simulink model "uav_1"  (R2015b)
settings: Solver=ode4  StartTime=0.0  StopTime=10  FixedStep=0.05  RelTol=1e-3
undefined symbols (not defined in the file): ctrsel, dphi_init, dpsi_init, dthe_init, dx_init, dy_init, dz_init, g, Jx, Jy, Jz, K1, K2, K3, K4, K5, K6, kt, l, m, omega1, omega2, omega3, omega4, phi_init, psi_init, the_init, x_init, y_init, z_init
settings Model: Creator=Administrator  LastModifiedBy=Administrator

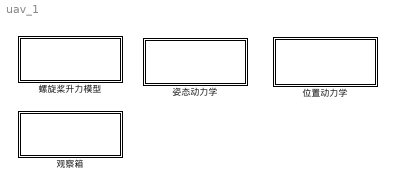
== system uav_1 ==
  位置动力学 : Subsystem
  姿态动力学 : Subsystem
  螺旋桨升力模型 : Subsystem
  观察箱 : Subsystem

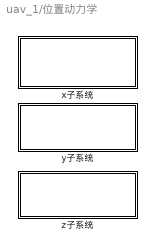
== system uav_1/位置动力学 ==
  x子系统 : Subsystem
  y子系统 : Subsystem
  z子系统 : Subsystem

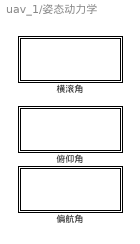
== system uav_1/姿态动力学 ==
  俯仰角 : Subsystem
  偏航角 : Subsystem
  横滚角 : Subsystem

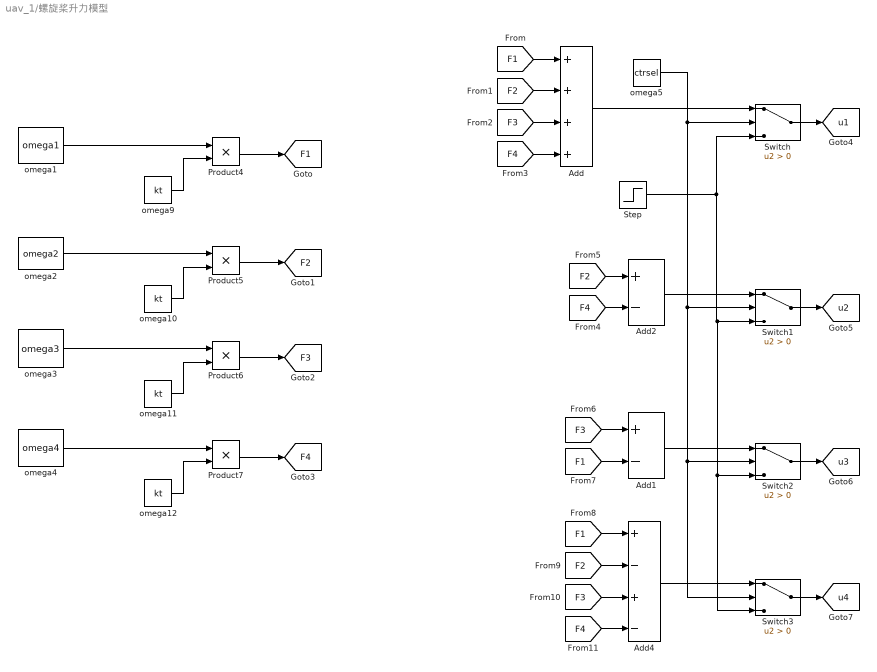
== system uav_1/螺旋桨升力模型 ==
  Add : Sum  Inputs=++++
  Add1 : Sum  Inputs=+-
  Add2 : Sum  Inputs=+-
  Add4 : Sum  Inputs=+-+-
  Product{4..7} (4 alike) : Product
  Step : Step  After=400  SampleTime=0
  Switch{,1..3} (4 alike) : Switch  Criteria=u2 > Threshold
  omega1 : Constant  Value=omega1
  omega{9..12} (4 alike) : Constant  Value=kt
  omega2 : Constant  Value=omega2
  omega3 : Constant  Value=omega3
  omega4 : Constant  Value=omega4
  omega5 : Constant  Value=ctrsel
  tag scope: F1=global, F2=global, F3=global, F4=global, u1=global, u2=global, u3=global, u4=global
  wires:
  [F3] -> Add/3
  [F4] -> Add/4
  [F1] -> Add1/2
  [F3] -> Add1/1
  [F2] -> Add/2
  [F1] -> Add/1
  [F1] -> Add4/1
  [F2] -> Add4/2
  [F3] -> Add4/3
  [F4] -> Add4/4
  [F4] -> Add2/2
  [F2] -> Add2/1
  omega1/1 -> Product4/1
  omega9/1 -> Product4/2
  Product4/1 -> [F1]
  omega2/1 -> Product5/1
  omega10/1 -> Product5/2
  Product5/1 -> [F2]
  omega3/1 -> Product6/1
  omega11/1 -> Product6/2
  Product6/1 -> [F3]
  omega4/1 -> Product7/1
  omega12/1 -> Product7/2
  Product7/1 -> [F4]
  omega5/1 -> Switch/2, Switch1/2, Switch2/2, Switch3/2
  Step/1 -> Switch/3, Switch3/3, Switch2/3, Switch1/3
  Add/1 -> Switch/1
  Add2/1 -> Switch1/1
  Add1/1 -> Switch2/1
  Add4/1 -> Switch3/1
  Switch/1 -> [u1]
  Switch1/1 -> [u2]
  Switch2/1 -> [u3]
  Switch3/1 -> [u4]

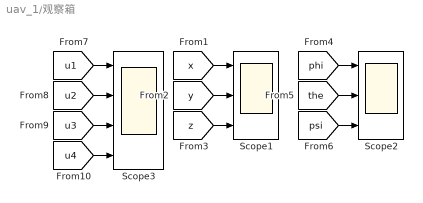
== system uav_1/观察箱 ==
  Scope1 : Scope  NumInputPorts=3
  Scope2 : Scope  NumInputPorts=3
  Scope3 : Scope  NumInputPorts=4
  wires:
  [x] -> Scope1/1
  [y] -> Scope1/2
  [z] -> Scope1/3
  [phi] -> Scope2/1
  [the] -> Scope2/2
  [psi] -> Scope2/3
  [u1] -> Scope3/1
  [u2] -> Scope3/2
  [u3] -> Scope3/3
  [u4] -> Scope3/4

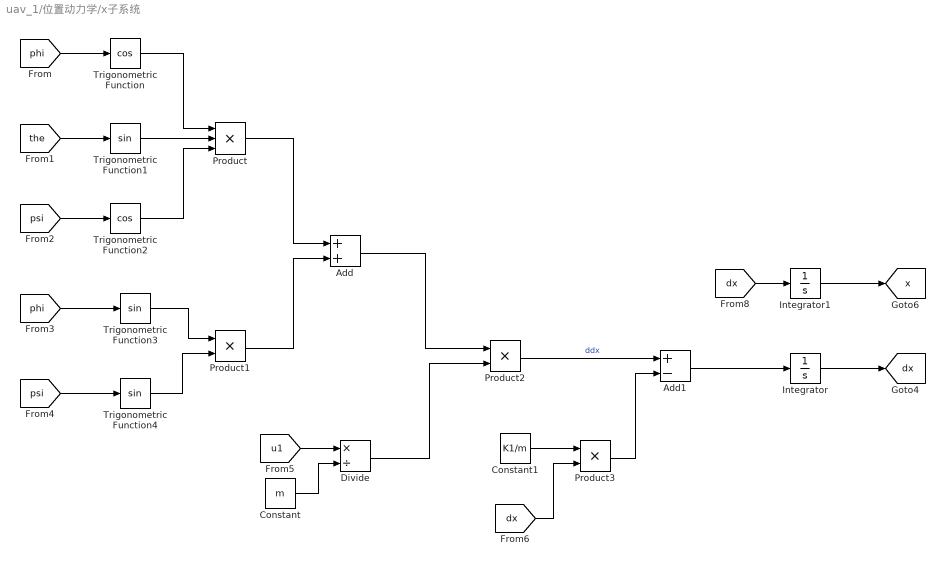
== system uav_1/位置动力学/x子系统 ==
  Add : Sum
  Add1 : Sum  Inputs=+-
  Constant : Constant  Value=m
  Constant1 : Constant  Value=K1/m
  Divide : Product  Inputs=*/
  Integrator : Integrator  InitialCondition=dx_init
  Integrator1 : Integrator  InitialCondition=x_init
  Product : Product  Inputs=3
  Product1 : Product
  Product2 : Product
  Product3 : Product
  Trigonometric Function : Trigonometry  Operator=cos
  Trigonometric Function1 : Trigonometry
  Trigonometric Function2 : Trigonometry  Operator=cos
  Trigonometric Function3 : Trigonometry
  Trigonometric Function4 : Trigonometry
  tag scope: dx=global, x=global
  wires:
  [phi] -> Trigonometric Function/1
  [the] -> Trigonometric Function1/1
  [psi] -> Trigonometric Function2/1
  Trigonometric Function1/1 -> Product/2
  Trigonometric Function/1 -> Product/1
  Trigonometric Function2/1 -> Product/3
  [phi] -> Trigonometric Function3/1
  [psi] -> Trigonometric Function4/1
  Trigonometric Function3/1 -> Product1/1
  Trigonometric Function4/1 -> Product1/2
  Product/1 -> Add/1
  Product1/1 -> Add/2
  [u1] -> Divide/1
  Constant/1 -> Divide/2
  Add/1 -> Product2/1
  Divide/1 -> Product2/2
  Product2/1 -> Add1/1  "ddx"
  Constant1/1 -> Product3/1
  Add1/1 -> Integrator/1
  Product3/1 -> Add1/2
  [dx] -> Product3/2
  Integrator/1 -> [dx]
  [dx] -> Integrator1/1
  Integrator1/1 -> [x]

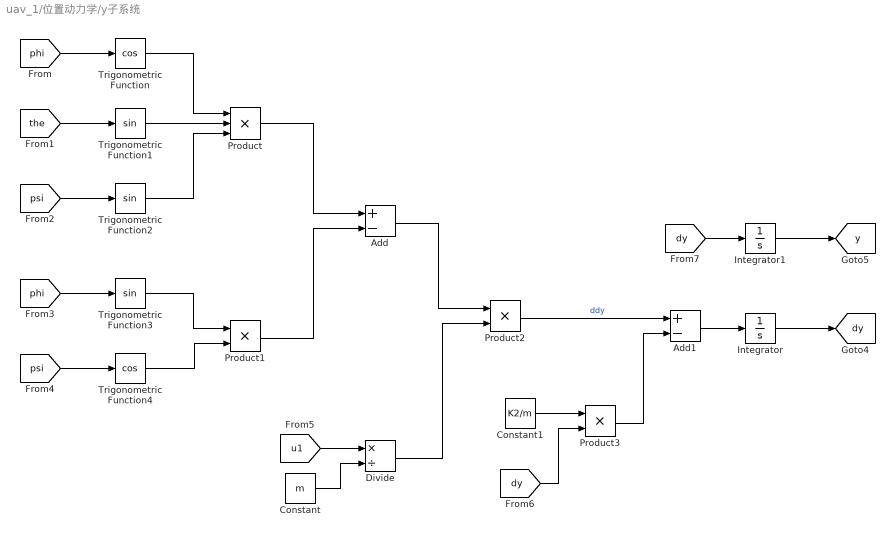
== system uav_1/位置动力学/y子系统 ==
  Add : Sum  Inputs=+-
  Add1 : Sum  Inputs=+-
  Constant : Constant  Value=m
  Constant1 : Constant  Value=K2/m
  Divide : Product  Inputs=*/
  Integrator : Integrator  InitialCondition=dy_init
  Integrator1 : Integrator  InitialCondition=y_init
  Product : Product  Inputs=3
  Product1 : Product
  Product2 : Product
  Product3 : Product
  Trigonometric Function : Trigonometry  Operator=cos
  Trigonometric Function1 : Trigonometry
  Trigonometric Function2 : Trigonometry
  Trigonometric Function3 : Trigonometry
  Trigonometric Function4 : Trigonometry  Operator=cos
  tag scope: dy=global, y=global
  wires:
  [phi] -> Trigonometric Function/1
  [the] -> Trigonometric Function1/1
  [psi] -> Trigonometric Function2/1
  Trigonometric Function1/1 -> Product/2
  Trigonometric Function/1 -> Product/1
  Trigonometric Function2/1 -> Product/3
  [phi] -> Trigonometric Function3/1
  [psi] -> Trigonometric Function4/1
  Trigonometric Function3/1 -> Product1/1
  Trigonometric Function4/1 -> Product1/2
  Product/1 -> Add/1
  Product1/1 -> Add/2
  [u1] -> Divide/1
  Constant/1 -> Divide/2
  Add/1 -> Product2/1
  Divide/1 -> Product2/2
  Constant1/1 -> Product3/1
  [dy] -> Product3/2
  Product2/1 -> Add1/1  "ddy"
  Product3/1 -> Add1/2
  Add1/1 -> Integrator/1
  Integrator/1 -> [dy]
  [dy] -> Integrator1/1
  Integrator1/1 -> [y]

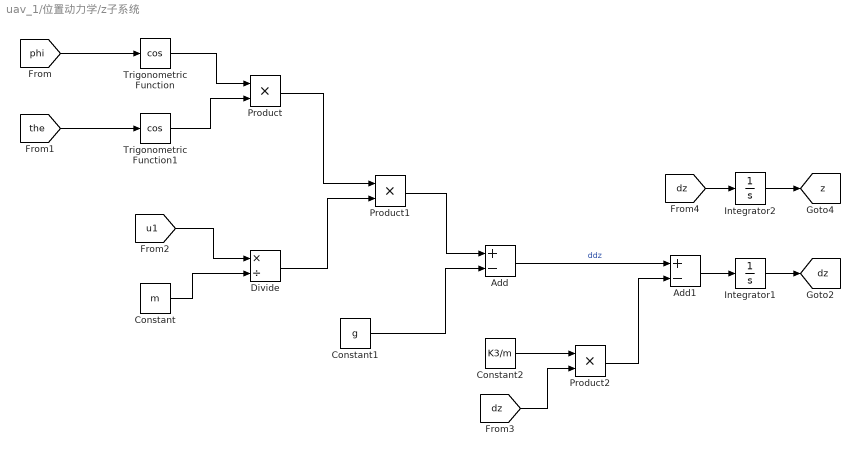
== system uav_1/位置动力学/z子系统 ==
  Add : Sum  Inputs=+-
  Add1 : Sum  Inputs=+-
  Constant : Constant  Value=m
  Constant1 : Constant  Value=g
  Constant2 : Constant  Value=K3/m
  Divide : Product  Inputs=*/
  Integrator1 : Integrator  InitialCondition=dz_init
  Integrator2 : Integrator  InitialCondition=z_init
  Product : Product
  Product1 : Product
  Product2 : Product
  Trigonometric Function : Trigonometry  Operator=cos
  Trigonometric Function1 : Trigonometry  Operator=cos
  tag scope: dz=global, z=global
  wires:
  [phi] -> Trigonometric Function/1
  [the] -> Trigonometric Function1/1
  Trigonometric Function/1 -> Product/1
  Trigonometric Function1/1 -> Product/2
  [u1] -> Divide/1
  Constant/1 -> Divide/2
  Product/1 -> Product1/1
  Divide/1 -> Product1/2
  Product1/1 -> Add/1
  Constant1/1 -> Add/2
  Add/1 -> Add1/1  "ddz"
  Constant2/1 -> Product2/1
  Product2/1 -> Add1/2
  Add1/1 -> Integrator1/1
  [dz] -> Product2/2
  Integrator1/1 -> [dz]
  [dz] -> Integrator2/1
  Integrator2/1 -> [z]

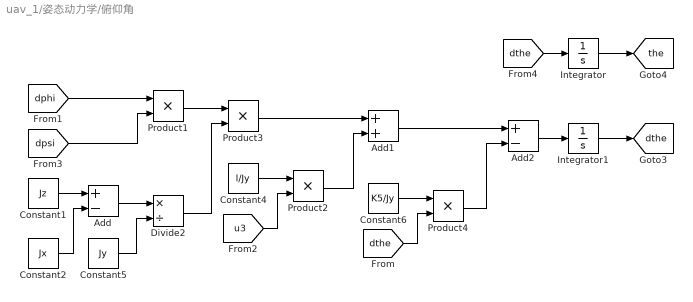
== system uav_1/姿态动力学/俯仰角 ==
  Add : Sum  Inputs=+-
  Add1 : Sum
  Add2 : Sum  Inputs=+-
  Constant1 : Constant  Value=Jz
  Constant2 : Constant  Value=Jx
  Constant4 : Constant  Value=l/Jy
  Constant5 : Constant  Value=Jy
  Constant6 : Constant  Value=K5/Jy
  Divide2 : Product  Inputs=*/
  Integrator : Integrator  InitialCondition=the_init
  Integrator1 : Integrator  InitialCondition=dthe_init
  Product{1..4} (4 alike) : Product
  tag scope: dthe=global, the=global
  wires:
  Constant4/1 -> Product2/1
  [u3] -> Product2/2
  [dphi] -> Product1/1
  [dpsi] -> Product1/2
  Constant1/1 -> Add/1
  Constant2/1 -> Add/2
  Add/1 -> Divide2/1
  Constant5/1 -> Divide2/2
  Product1/1 -> Product3/1
  Divide2/1 -> Product3/2
  Product3/1 -> Add1/1
  Product2/1 -> Add1/2
  Constant6/1 -> Product4/1
  [dthe] -> Product4/2
  Product4/1 -> Add2/2
  Add1/1 -> Add2/1
  Add2/1 -> Integrator1/1
  Integrator1/1 -> [dthe]
  [dthe] -> Integrator/1
  Integrator/1 -> [the]

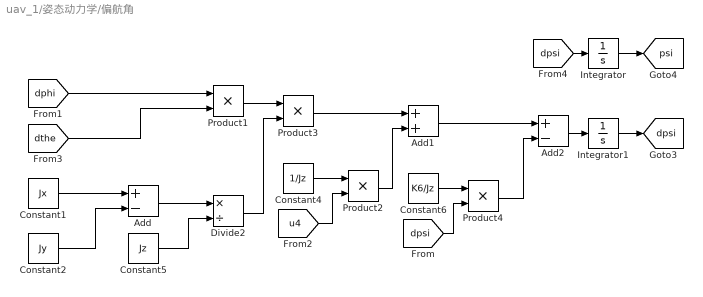
== system uav_1/姿态动力学/偏航角 ==
  Add : Sum  Inputs=+-
  Add1 : Sum
  Add2 : Sum  Inputs=+-
  Constant1 : Constant  Value=Jx
  Constant2 : Constant  Value=Jy
  Constant4 : Constant  Value=1/Jz
  Constant5 : Constant  Value=Jz
  Constant6 : Constant  Value=K6/Jz
  Divide2 : Product  Inputs=*/
  Integrator : Integrator  InitialCondition=psi_init
  Integrator1 : Integrator  InitialCondition=dpsi_init
  Product{1..4} (4 alike) : Product
  tag scope: dpsi=global, psi=global
  wires:
  Constant4/1 -> Product2/1
  [u4] -> Product2/2
  [dphi] -> Product1/1
  [dthe] -> Product1/2
  Constant1/1 -> Add/1
  Constant2/1 -> Add/2
  Add/1 -> Divide2/1
  Constant5/1 -> Divide2/2
  Product1/1 -> Product3/1
  Divide2/1 -> Product3/2
  Product3/1 -> Add1/1
  Product2/1 -> Add1/2
  Constant6/1 -> Product4/1
  [dpsi] -> Product4/2
  Product4/1 -> Add2/2
  Add1/1 -> Add2/1
  Add2/1 -> Integrator1/1
  Integrator1/1 -> [dpsi]
  [dpsi] -> Integrator/1
  Integrator/1 -> [psi]

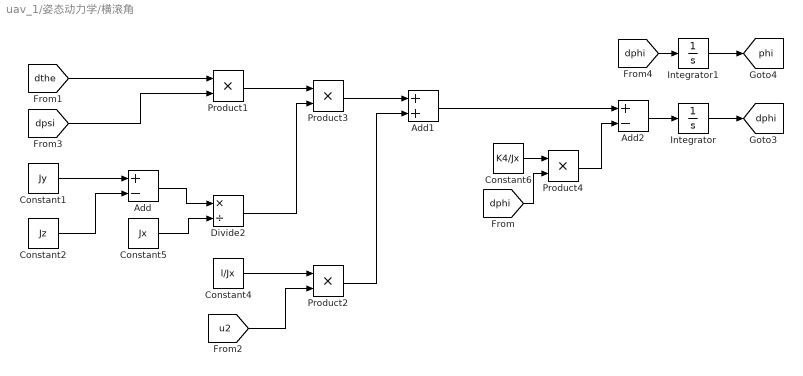
== system uav_1/姿态动力学/横滚角 ==
  Add : Sum  Inputs=+-
  Add1 : Sum
  Add2 : Sum  Inputs=+-
  Constant1 : Constant  Value=Jy
  Constant2 : Constant  Value=Jz
  Constant4 : Constant  Value=l/Jx
  Constant5 : Constant  Value=Jx
  Constant6 : Constant  Value=K4/Jx
  Divide2 : Product  Inputs=*/
  Integrator : Integrator  InitialCondition=dphi_init
  Integrator1 : Integrator  InitialCondition=phi_init
  Product{1..4} (4 alike) : Product
  tag scope: dphi=global, phi=global
  wires:
  Integrator/1 -> [dphi]
  [u2] -> Product2/2
  Constant4/1 -> Product2/1
  [dthe] -> Product1/1
  [dpsi] -> Product1/2
  Constant1/1 -> Add/1
  Constant2/1 -> Add/2
  Add/1 -> Divide2/1
  Constant5/1 -> Divide2/2
  Product1/1 -> Product3/1
  Divide2/1 -> Product3/2
  Product3/1 -> Add1/1
  Product2/1 -> Add1/2
  Add1/1 -> Add2/1
  Constant6/1 -> Product4/1
  [dphi] -> Product4/2
  Product4/1 -> Add2/2
  Add2/1 -> Integrator/1
  [dphi] -> Integrator1/1
  Integrator1/1 -> [phi]
